simulink model "21-E"  (R2014a)
settings: Solver=FixedStepDiscrete  StartTime=0.0  StopTime=10.0  FixedStep=0.0005  RelTol=1e-3
undefined symbols (not defined in the file): add_k1_100, add_k2_100, ADDspeed, cal_acc_div, cal_acc_flo_add, cal_acc_min, cal_an_div, cal_an_min, cal_bre_div, cal_bre_en_add, cal_bre_flo_add, cal_bre_min, cal_conf_off, cal_conf_on, controller, ecucoder_acal, enres_on_add, enres_per_add
libraries: simulink x165, ec55xxlib x29
(part 6 of 6)

== system 21-E/run/ctrl/Subsystem1/control/Subsystem6 ==
  x1 : Inport
  x2 : Inport  Port=2
  x3 : Inport  Port=3
  x4 : Inport  Port=4
  k1 : Inport  Port=5
  k2 : Inport  Port=6
  Subsystem4 : Subsystem
  Subsystem5 : Subsystem
  alp1d : Outport
  alp2d : Outport  Port=2
  wires:
  Subsystem5/1(alp2d) -> alp2d/1
  x4/1 -> Subsystem5/2(x4)
  x2/1 -> Subsystem5/1(x2)
  k2/1 -> Subsystem5/3(k2)
  x3/1 -> Subsystem4/2(x3)
  k1/1 -> Subsystem4/3(k1)
  x1/1 -> Subsystem4/1(x1)
  Subsystem4/1(alp1d) -> alp1d/1

== system 21-E/run/ctrl/amk_tpostive1/差速/Subsystem1 ==
  vy : Inport
  yaw : Inport  Port=2
  ax : Inport  Port=3
  ay : Inport  Port=4
  Data Store Read : DataStoreRead  DataStoreName=ANGLE
  Data Store Read1 : DataStoreRead  DataStoreName=Vture
  Fz : Subsystem
  K : MATLAB Function  TreatAsAtomicUnit=on
  K1 : MATLAB Function  TreatAsAtomicUnit=on
  K2 : MATLAB Function  TreatAsAtomicUnit=on
  K3 : MATLAB Function  TreatAsAtomicUnit=on
  alp : Subsystem
  ctrl : Subsystem
  u3 : Outport
  w1 : Outport  Port=2
  w2 : Outport  Port=3
  w3 : Outport  Port=4
  w4 : Outport  Port=5
  tag scope: alp1l=global, alp1r=global, alp2l=global, alp2r=global, del=global, k1l=global, k1r=global, k2l=global, k2r=global, vx=global, vy=global, yaw=global
  wires:
  K3/1(k) -> [k2r]
  Fz/4(W2r) -> w4/1, K3/1(w)
  K2/1(k) -> [k2l]
  Fz/3(W2l) -> w3/1, K2/1(w)
  K1/1(k) -> [k1r]
  Fz/2(W1r) -> w2/1, K1/1(w)
  K/1(k) -> [k1l]
  Fz/1(W1l) -> w1/1, K/1(w)
  ay/1 -> Fz/2(ay)
  ax/1 -> Fz/1(ax)
  alp/4(alp_2R) -> [alp2r]
  alp/3(alp_2L) -> [alp2l]
  alp/2(alp_1R) -> [alp1r]
  alp/1(alp_1L) -> [alp1l]
  vy/1 -> [vy]
  yaw/1 -> [yaw]
  ctrl/1(u3) -> u3/1
  Data Store Read/1 -> [del]
  Data Store Read1/1 -> [vx]

== system 21-E/run/ctrl/amk_tpostive1/差速/Subsystem2 ==
  vx : Inport
  an : Inport  Port=2
  Add : Sum  Inputs=+-
  Add1 : Sum  Inputs=+-
  Add2 : Sum  Inputs=+-
  Constant : Constant  Value=0.01
  Constant1 : Constant  Value=0.01
  Constant2 : Constant  Value=0.01
  Delay : Delay  DelayLength=1  InitialCondition=0
  Delay1 : Delay  DelayLength=1  InitialCondition=0
  Delay2 : Delay  DelayLength=1  InitialCondition=0
  Product{,1..3} (4 alike) : Product  Inputs=*/
  Subsystem : Subsystem
  Trigonometric Function : Trigonometry  Operator=atan
  vy : Outport
  yaw : Outport  Port=2
  ax : Outport  Port=3
  ay : Outport  Port=4
  wires:
  Product/1 -> ay/1
  Add/1 -> Product/1
  Constant/1 -> Product/2
  Add1/1 -> Product1/1
  Constant1/1 -> Product1/2
  Product1/1 -> ax/1
  Delay1/1 -> Add1/2
  Delay/1 -> Add/2
  Subsystem/1(vy) -> Product3/1, vy/1, Delay/1, Add/1
  an/1 -> Subsystem/1(angle)
  vx/1 -> Product3/2, Delay1/1, Add1/1
  Add2/1 -> Product2/1
  Constant2/1 -> Product2/2
  Delay2/1 -> Add2/2
  Trigonometric Function/1 -> Add2/1, Delay2/1
  Product3/1 -> Trigonometric Function/1
  Product2/1 -> yaw/1

== system 21-E/run/ctrl/amk_tpostive1/限滑/V前 ==
  Data Store Read : DataStoreRead  DataStoreName=V1
  Data Store Read1 : DataStoreRead  DataStoreName=V2
  MinMax : MinMax  Function=max  Inputs=2
  Out1 : Outport
  wires:
  MinMax/1 -> Out1/1
  Data Store Read/1 -> MinMax/1
  Data Store Read1/1 -> MinMax/2

== system 21-E/run/ctrl/amk_tpostive1/限滑/V后 ==
  Data Store Read2 : DataStoreRead  DataStoreName=V3
  Data Store Read3 : DataStoreRead  DataStoreName=V4
  MinMax : MinMax  Function=max  Inputs=2
  Out1 : Outport
  wires:
  MinMax/1 -> Out1/1
  Data Store Read2/1 -> MinMax/1
  Data Store Read3/1 -> MinMax/2

== system 21-E/run/ctrl/amk_tpostive1/限滑/扭矩*PI1 ==
  扭矩 : Inport
  滑移率输入 : Inport  Port=2
  Constant2 : Constant
  Constant8 : Constant  Value=0.2
  Product : Product
  Saturation1 : Saturate  UpperLimit=1  LowerLimit=0
  Saturation2 : Saturate  UpperLimit=1  LowerLimit=0
  Saturation3 : Saturate  UpperLimit=1  LowerLimit=-1
  Saturation6 : Saturate  UpperLimit=2000  LowerLimit=0
  Sum1 : Sum  Inputs=|+-
  Sum4 : Sum  Inputs=|-+
  pid_discrete : Subsystem
  Out1 : Outport
  wires:
  Constant8/1 -> Sum4/2
  扭矩/1 -> Product/2
  Product/1 -> Saturation6/1
  Saturation6/1 -> Out1/1
  Saturation2/1 -> Product/1
  Saturation1/1 -> pid_discrete/2(y), Sum4/1
  Sum1/1 -> Saturation2/1
  Constant2/1 -> Sum1/1
  Sum4/1 -> Saturation3/1
  滑移率输入/1 -> Saturation1/1
  Saturation3/1 -> pid_discrete/1(err)
  pid_discrete/1(pid_out) -> Sum1/2  "pidhou"

== system 21-E/run/ctrl/amk_tpostive1/限滑/扭矩*PI2 ==
  滑移率输入 : Inport
  扭矩 : Inport  Port=2
  Constant2 : Constant
  Constant8 : Constant  Value=0.2
  Product : Product
  Saturation1 : Saturate  UpperLimit=1  LowerLimit=0
  Saturation2 : Saturate  UpperLimit=1  LowerLimit=0
  Saturation3 : Saturate  UpperLimit=1  LowerLimit=-1
  Saturation6 : Saturate  UpperLimit=2000  LowerLimit=0
  Sum1 : Sum  Inputs=|+-
  Sum4 : Sum  Inputs=|-+
  pid_discrete : Subsystem
  Out1 : Outport
  wires:
  扭矩/1 -> Product/2
  pid_discrete/1(pid_out) -> Sum1/2  "pidqian"
  Product/1 -> Saturation6/1
  Saturation6/1 -> Out1/1
  Saturation2/1 -> Product/1
  Saturation1/1 -> pid_discrete/2(y), Sum4/1
  Sum1/1 -> Saturation2/1
  Constant2/1 -> Sum1/1
  Sum4/1 -> Saturation3/1
  滑移率输入/1 -> Saturation1/1
  Constant8/1 -> Sum4/2
  Saturation3/1 -> pid_discrete/1(err)

== system 21-E/run/ctrl/amk_tpostive1/限滑/滑移率计算 ==
  V后 : Inport
  Add : Sum  Inputs=-+
  Constant : Constant  Value=0
  Data Store Read2 : DataStoreRead  DataStoreName=Vture
  Product1 : Product  Inputs=*/
  Switch2 : Switch  Criteria=u2 > Threshold  Threshold=500*1.88e-3
  Out : Outport
  wires:
  Data Store Read2/1 -> Add/1
  V后/1 -> Add/2, Switch2/2, Product1/2
  Add/1 -> Product1/1
  Product1/1 -> Switch2/1
  Constant/1 -> Switch2/3
  Switch2/1 -> Out/1

== system 21-E/run/ctrl/amk_tpostive1/限滑/滑移率计算1 ==
  V前 : Inport
  Add : Sum  Inputs=-+
  Constant : Constant  Value=0
  Data Store Read2 : DataStoreRead  DataStoreName=Vture
  Product1 : Product  Inputs=*/
  Switch2 : Switch  Criteria=u2 > Threshold  Threshold=500*1.88e-3
  Out : Outport
  wires:
  Data Store Read2/1 -> Add/1
  V前/1 -> Add/2, Switch2/2, Product1/2
  Add/1 -> Product1/1
  Product1/1 -> Switch2/1
  Constant/1 -> Switch2/3
  Switch2/1 -> Out/1

== system 21-E/run/ctrl/control/Subsystem6/Subsystem4 ==
  x1 : Inport
  x3 : Inport  Port=2
  k1 : Inport  Port=3
  Add : Sum  Inputs=+-
  Add1 : Sum  Inputs=+-
  Constant : Constant  Value=0.001
  Constant1 : Constant  Value=0.8
  Data Store Read : DataStoreRead  DataStoreName=a
  Divide : Product  Inputs=/*
  Gain : Gain  Gain=0.225
  Product : Product  Inputs=3
  Switch : Switch  Criteria=u2 > Threshold
  alp1d : Outport
  wires:
  Add/1 -> Product/2
  Add1/1 -> Divide/2
  Product/1 -> Add1/2
  Divide/1 -> alp1d/1
  Data Store Read/1 -> Add1/1
  Switch/1 -> Gain/1
  Constant/1 -> Switch/3
  x1/1 -> Product/3
  Constant1/1 -> Add/1
  Gain/1 -> Divide/1
  x3/1 -> Add/2, Switch/1, Switch/2
  k1/1 -> Product/1

== system 21-E/run/ctrl/control/Subsystem6/Subsystem5 ==
  x2 : Inport
  x4 : Inport  Port=2
  k2 : Inport  Port=3
  Add : Sum  Inputs=+-
  Add1 : Sum  Inputs=+-
  Constant : Constant  Value=0.001
  Constant1 : Constant  Value=0.8
  Data Store Read : DataStoreRead  DataStoreName=a
  Divide : Product  Inputs=/*
  Gain : Gain  Gain=0.225
  Product : Product  Inputs=3
  Switch : Switch  Criteria=u2 > Threshold
  alp2d : Outport
  wires:
  k2/1 -> Product/1
  x4/1 -> Switch/2, Switch/1, Add/2
  Gain/1 -> Divide/1
  Constant1/1 -> Add/1
  x2/1 -> Product/3
  Constant/1 -> Switch/3
  Switch/1 -> Gain/1
  Data Store Read/1 -> Add1/1
  Divide/1 -> alp2d/1
  Product/1 -> Add1/2
  Add1/1 -> Divide/2
  Add/1 -> Product/2

== system 21-E/run/ctrl/Subsystem1/control/Subsystem6/Subsystem4 ==
  x1 : Inport
  x3 : Inport  Port=2
  k1 : Inport  Port=3
  Add : Sum  Inputs=+-
  Add1 : Sum  Inputs=+-
  Constant : Constant  Value=0.001
  Constant1 : Constant  Value=0.8
  Data Store Read : DataStoreRead  DataStoreName=a
  Divide : Product  Inputs=/*
  Gain : Gain  Gain=0.225
  Product : Product  Inputs=3
  Switch : Switch  Criteria=u2 > Threshold
  alp1d : Outport
  wires:
  Add/1 -> Product/2
  Add1/1 -> Divide/2
  Product/1 -> Add1/2
  Divide/1 -> alp1d/1
  Data Store Read/1 -> Add1/1
  Switch/1 -> Gain/1
  Constant/1 -> Switch/3
  x1/1 -> Product/3
  Constant1/1 -> Add/1
  Gain/1 -> Divide/1
  x3/1 -> Add/2, Switch/1, Switch/2
  k1/1 -> Product/1

== system 21-E/run/ctrl/Subsystem1/control/Subsystem6/Subsystem5 ==
  x2 : Inport
  x4 : Inport  Port=2
  k2 : Inport  Port=3
  Add : Sum  Inputs=+-
  Add1 : Sum  Inputs=+-
  Constant : Constant  Value=0.001
  Constant1 : Constant  Value=0.8
  Data Store Read : DataStoreRead  DataStoreName=a
  Divide : Product  Inputs=/*
  Gain : Gain  Gain=0.225
  Product : Product  Inputs=3
  Switch : Switch  Criteria=u2 > Threshold
  alp2d : Outport
  wires:
  k2/1 -> Product/1
  x4/1 -> Switch/2, Switch/1, Add/2
  Gain/1 -> Divide/1
  Constant1/1 -> Add/1
  x2/1 -> Product/3
  Constant/1 -> Switch/3
  Switch/1 -> Gain/1
  Data Store Read/1 -> Add1/1
  Divide/1 -> alp2d/1
  Product/1 -> Add1/2
  Add1/1 -> Divide/2
  Add/1 -> Product/2

== system 21-E/run/ctrl/amk_tpostive1/差速/Subsystem1/Fz ==
  ax : Inport
  ay : Inport  Port=2
  Add : Sum
  L1 : Constant  Value=0.765
  L2 : Constant  Value=0.765
  M : Constant  Value=308
  Product : Product  Inputs=*/
  Subsystem : Subsystem
  Subsystem1 : Subsystem
  W1l : Outport
  W1r : Outport  Port=2
  W2l : Outport  Port=3
  W2r : Outport  Port=4
  wires:
  Subsystem1/2(w2r) -> W2r/1
  Subsystem1/1(w2l) -> W2l/1
  Subsystem/2(w1r) -> W1r/1
  Subsystem/1(w1l) -> W1l/1
  [ay] -> Subsystem1/4(ay)
  [ay] -> Subsystem/4(ay)
  [ax] -> Subsystem1/3(ax)
  [ax] -> Subsystem/3(ax)
  [L2] -> Subsystem/2(L2)
  Product/1 -> Subsystem/1(fac), Subsystem1/1(fac)
  [L1] -> Subsystem1/2(L1)
  ay/1 -> [ay]
  ax/1 -> [ax]
  M/1 -> Product/1
  Add/1 -> Product/2
  L2/1 -> Add/2, [L2]
  L1/1 -> Add/1, [L1]

== system 21-E/run/ctrl/amk_tpostive1/差速/Subsystem1/alp ==
  Constant{,2,4,6} (4 alike) : Constant  Value=0.765
  Constant{1,3,5,7} (4 alike) : Constant  Value=1.16
  MATLAB Function1 : MATLAB Function  TreatAsAtomicUnit=on
  MATLAB Function2 : MATLAB Function  TreatAsAtomicUnit=on
  MATLAB Function3 : MATLAB Function  TreatAsAtomicUnit=on
  MATLAB Function4 : MATLAB Function  TreatAsAtomicUnit=on
  Saturation{,1..3} (4 alike) : Saturate  UpperLimit=9/180*pi  LowerLimit=0
  alp_1L : Outport
  alp_1R : Outport  Port=2
  alp_2L : Outport  Port=3
  alp_2R : Outport  Port=4
  wires:
  Saturation3/1 -> alp_1L/1
  Saturation2/1 -> alp_2R/1
  Saturation1/1 -> alp_2L/1
  Saturation/1 -> alp_1R/1
  Constant6/1 -> MATLAB Function1/5(L1)
  Constant7/1 -> MATLAB Function1/6(D)
  Constant5/1 -> MATLAB Function4/5(D)
  Constant4/1 -> MATLAB Function4/4(L2)
  Constant2/1 -> MATLAB Function3/4(L2)
  Constant3/1 -> MATLAB Function3/5(D)
  Constant1/1 -> MATLAB Function2/6(D)
  MATLAB Function2/1(alp_1R) -> Saturation/1
  MATLAB Function4/1(alp_2R) -> Saturation2/1
  [vy] -> MATLAB Function1/2(vy)
  [yaw] -> MATLAB Function4/3(yaw)
  [del] -> MATLAB Function1/4(del)
  [vy] -> MATLAB Function2/2(vy)
  [del] -> MATLAB Function2/4(del)
  [vx] -> MATLAB Function2/1(v)
  MATLAB Function1/1(alp_1L) -> Saturation3/1
  [yaw] -> MATLAB Function3/3(yaw)
  [vx] -> MATLAB Function1/1(v)
  [yaw] -> MATLAB Function1/3(yaw)
  [vx] -> MATLAB Function4/1(v)
  [vy] -> MATLAB Function3/2(vy)
  [yaw] -> MATLAB Function2/3(yaw)
  MATLAB Function3/1(alp_2L) -> Saturation1/1
  [vy] -> MATLAB Function4/2(vy)
  Constant/1 -> MATLAB Function2/5(L1)
  [vx] -> MATLAB Function3/1(v)

== system 21-E/run/ctrl/amk_tpostive1/差速/Subsystem1/ctrl ==
  Manual Switch2 : ManualSwitch  CurrentSetting=0
  PID : Subsystem
  Subsystem1 : Subsystem
  rho : Subsystem
  slide : Subsystem
  u3 : Outport
  tag scope: e3=global, xd3=global
  wires:
  Manual Switch2/1 -> u3/1
  slide/1(u3) -> Manual Switch2/2
  PID/1(pid3) -> Manual Switch2/1
  rho/1(rho3) -> slide/3(rho3)
  [xd3] -> slide/2(x3)
  [e3] -> slide/1(e3)
  [yaw] -> PID/2(y3)
  [e3] -> PID/1(err3)
  Subsystem1/2(xd3) -> [xd3]
  Subsystem1/1(e3) -> [e3]
  [del] -> Subsystem1/3(del)
  [yaw] -> Subsystem1/2(yaw)
  [vx] -> Subsystem1/1(v)

== system 21-E/run/ctrl/amk_tpostive1/差速/Subsystem2/Subsystem ==
  angle : Inport
  Add : Sum
  Data Store Read2 : DataStoreRead  DataStoreName=V1
  Data Store Read3 : DataStoreRead  DataStoreName=V2
  Gain : Gain  Gain=0.5
  Product : Product
  Product1 : Product
  Trigonometric Function : Trigonometry
  Trigonometric Function1 : Trigonometry
  vy : Outport
  wires:
  Product/1 -> Add/1
  Trigonometric Function/1 -> Product/2
  Product1/1 -> Add/2
  Data Store Read3/1 -> Product1/1
  Data Store Read2/1 -> Product/1
  Add/1 -> Gain/1
  angle/1 -> Trigonometric Function1/1, Trigonometric Function/1
  Gain/1 -> vy/1
  Trigonometric Function1/1 -> Product1/2

== system 21-E/run/ctrl/amk_tpostive1/限滑/扭矩*PI1/pid_discrete ==
  err : Inport
  y : Inport  Port=2
  Add : Sum  Inputs=4
  Constant : Constant  Value=0.01
  Constant1 : Constant  Value=0.6
  Constant10 : Constant  Value=0
  Constant2 : Constant  Value=0.15
  Constant3 : Constant  Value=0.03
  Constant4 : Constant  Value=0.07
  Constant5 : Constant  Value=0
  Constant6 : Constant  Value=2000
  Constant7 : Constant  Value=0.6
  Constant8 : Constant  Value=0.03
  Constant9 : Constant  Value=0.01
  D : Subsystem
  I : Subsystem
  Memory : Memory  InheritSampleTime=on
  P : Subsystem
  dead_zone : Subsystem
  pid_out : Outport
  wires:
  Constant/1 -> dead_zone/2(err0)
  err/1 -> dead_zone/1(err_in)
  Add/1 -> pid_out/1, Memory/1
  Memory/1 -> Add/4, I/2(pid_in)
  P/1(Up) -> Add/1
  I/1(Ui) -> Add/2
  dead_zone/1(err_out) -> P/1(err), D/2(err), I/1(err)
  D/1(Ude) -> Add/3
  Constant1/1 -> P/2(kp)
  Constant4/1 -> I/5(ki)
  Constant6/1 -> I/7(up)
  Constant5/1 -> I/6(down)
  Constant2/1 -> I/3(sep)
  Constant3/1 -> I/4(len)
  y/1 -> D/1(y)
  Constant7/1 -> D/3(kp)
  Constant8/1 -> D/4(Td)
  Constant10/1 -> D/6(gama), D/7(zero)
  Constant9/1 -> D/5(T)

== system 21-E/run/ctrl/amk_tpostive1/限滑/扭矩*PI2/pid_discrete ==
  err : Inport
  y : Inport  Port=2
  Add : Sum  Inputs=4
  Constant : Constant  Value=0.01
  Constant1 : Constant  Value=0.6
  Constant10 : Constant  Value=0
  Constant2 : Constant  Value=0.15
  Constant3 : Constant  Value=0.03
  Constant4 : Constant  Value=0.07
  Constant5 : Constant  Value=0
  Constant6 : Constant  Value=2000
  Constant7 : Constant  Value=0.6
  Constant8 : Constant  Value=0.03
  Constant9 : Constant  Value=0.01
  D : Subsystem
  I : Subsystem
  Memory : Memory  InheritSampleTime=on
  P : Subsystem
  dead_zone : Subsystem
  pid_out : Outport
  wires:
  Constant/1 -> dead_zone/2(err0)
  err/1 -> dead_zone/1(err_in)
  Add/1 -> pid_out/1, Memory/1
  Memory/1 -> Add/4, I/2(pid_in)
  P/1(Up) -> Add/1
  I/1(Ui) -> Add/2
  dead_zone/1(err_out) -> P/1(err), D/2(err), I/1(err)
  D/1(Ude) -> Add/3
  Constant1/1 -> P/2(kp)
  Constant4/1 -> I/5(ki)
  Constant6/1 -> I/7(up)
  Constant5/1 -> I/6(down)
  Constant2/1 -> I/3(sep)
  Constant3/1 -> I/4(len)
  y/1 -> D/1(y)
  Constant7/1 -> D/3(kp)
  Constant8/1 -> D/4(Td)
  Constant10/1 -> D/6(gama), D/7(zero)
  Constant9/1 -> D/5(T)

== system 21-E/run/ctrl/amk_tpostive1/差速/Subsystem1/Fz/Subsystem ==
  fac : Inport
  L2 : Inport  Port=2
  ax : Inport  Port=3
  ay : Inport  Port=4
  Add : Sum  Inputs=+-
  Add1 : Sum  Inputs=+-
  Add2 : Sum  Inputs=2
  D : Constant  Value=1.18
  Demux : Demux  Outputs=2
  Gain : Gain  Gain=0.5
  Mux : Mux  Inputs=2
  Product : Product  Inputs=**/
  Product1 : Product
  g : Gain  Gain=9.8
  h1 : Gain  Gain=0.269
  h2 : Gain  Gain=0.269
  w1l : Outport
  w1r : Outport  Port=2
  wires:
  Demux/2 -> w1r/1
  Demux/1 -> w1l/1
  Product1/1 -> Demux/1
  fac/1 -> Product1/1
  Mux/1 -> Product1/2
  Add2/1 -> Mux/2
  Add1/1 -> Mux/1
  Product/1 -> Add1/2, Add2/2
  Gain/1 -> Add1/1, Add2/1
  D/1 -> Product/3
  ay/1 -> Product/2
  h2/1 -> Product/1
  Add/1 -> Gain/1
  h1/1 -> Add/2
  g/1 -> Add/1
  ax/1 -> h1/1
  L2/1 -> g/1, h2/1

== system 21-E/run/ctrl/amk_tpostive1/差速/Subsystem1/Fz/Subsystem1 ==
  fac : Inport
  L1 : Inport  Port=2
  ax : Inport  Port=3
  ay : Inport  Port=4
  Add : Sum  Inputs=2
  Add1 : Sum  Inputs=+-
  Add2 : Sum  Inputs=2
  D : Constant  Value=1.16
  Demux : Demux  Outputs=2
  Gain : Gain  Gain=0.5
  Mux : Mux  Inputs=2
  Product : Product  Inputs=**/
  Product1 : Product
  g : Gain  Gain=9.8
  h1 : Gain  Gain=0.269
  h2 : Gain  Gain=0.269
  w2l : Outport
  w2r : Outport  Port=2
  wires:
  L1/1 -> h2/1, g/1
  ax/1 -> h1/1
  g/1 -> Add/1
  h1/1 -> Add/2
  Add/1 -> Gain/1
  h2/1 -> Product/1
  ay/1 -> Product/2
  D/1 -> Product/3
  Gain/1 -> Add2/1, Add1/1
  Product/1 -> Add2/2, Add1/2
  Add1/1 -> Mux/1
  Add2/1 -> Mux/2
  Mux/1 -> Product1/2
  fac/1 -> Product1/1
  Product1/1 -> Demux/1
  Demux/1 -> w2l/1
  Demux/2 -> w2r/1

== system 21-E/run/ctrl/amk_tpostive1/差速/Subsystem1/ctrl/PID ==
  err3 : Inport
  y3 : Inport  Port=2
  pid_continuous2 : Subsystem
  pid3 : Outport
  wires:
  pid_continuous2/1(pid_out) -> pid3/1
  y3/1 -> pid_continuous2/2(y)
  err3/1 -> pid_continuous2/1(err)

== system 21-E/run/ctrl/amk_tpostive1/差速/Subsystem1/ctrl/Subsystem1 ==
  v : Inport
  yaw : Inport  Port=2
  del : Inport  Port=3
  Add2 : Sum  Inputs=+-
  Add3 : Sum  Inputs=2
  Constant1 : Constant
  K : Constant  Value=0.0002
  L_1 : Gain  Gain=1/(0.765+0.765)
  Math Function : Math  Operator=square  SaturateOnIntegerOverflow=on
  Product : Product  Inputs=**/
  Product1 : Product
  e3 : Outport
  xd3 : Outport  Port=2
  wires:
  yaw/1 -> Add2/2
  Constant1/1 -> Add3/2
  Math Function/1 -> Product1/1
  L_1/1 -> Product/1
  del/1 -> L_1/1
  Product1/1 -> Add3/1
  Add3/1 -> Product/3
  v/1 -> Math Function/1, Product/2
  K/1 -> Product1/2
  Add2/1 -> e3/1
  Product/1 -> Add2/1, xd3/1

== system 21-E/run/ctrl/amk_tpostive1/差速/Subsystem1/ctrl/rho ==
  Subsystem3 : Subsystem
  rho3 : Outport
  wires:
  Subsystem3/1(rho3) -> rho3/1
  [k1l] -> Subsystem3/1(k1)
  [k1r] -> Subsystem3/2(k2)
  [k2l] -> Subsystem3/3(k3)
  [k2r] -> Subsystem3/4(k4)
  [vx] -> Subsystem3/5(v)
  [yaw] -> Subsystem3/6(yaw)
  [vy] -> Subsystem3/7(vy)
  [del] -> Subsystem3/8(del)

== system 21-E/run/ctrl/amk_tpostive1/差速/Subsystem1/ctrl/slide ==
  e3 : Inport
  x3 : Inport  Port=2
  rho3 : Inport  Port=3
  Add3 : Sum  Inputs=3
  Derivative2 : Derivative
  MATLAB Function2 : MATLAB Function  TreatAsAtomicUnit=on
  Product2 : Product
  k3 : Gain  Gain=5
  u3 : Outport
  wires:
  x3/1 -> Derivative2/1
  Derivative2/1 -> Add3/1
  rho3/1 -> Product2/2
  e3/1 -> MATLAB Function2/1(e), k3/1
  Product2/1 -> Add3/3
  k3/1 -> Add3/2
  MATLAB Function2/1(s) -> Product2/1
  Add3/1 -> u3/1

== system 21-E/run/ctrl/amk_tpostive1/限滑/扭矩*PI1/pid_discrete/D ==
  y : Inport
  err : Inport  Port=2
  kp : Inport  Port=3
  Td : Inport  Port=4
  T : Inport  Port=5
  gama : Inport  Port=6
  zero : Inport  Port=7
  Add{,1..3} (4 alike) : Sum  Inputs=-+
  From : From  Commented=on  GotoTag=dy
  From1 : From  Commented=on  GotoTag=dym
  MATLAB Function1 : MATLAB Function  TreatAsAtomicUnit=on
  MATLAB Function2 : MATLAB Function  Commented=on  TreatAsAtomicUnit=on
  Product : Product  Commented=on  Inputs=**/
  Unit Delay{,1,3..5} (5 alike) : UnitDelay  SampleTime=-1
  Unit Delay2 : UnitDelay  Commented=on  SampleTime=-1
  Ude : Outport
  Udy : Outport  Port=2
  wires:
  y/1 -> Unit Delay/1, Add/2
  Unit Delay/1 -> Unit Delay1/1, Add1/2, Add/1
  Add/1 -> [dy]
  Unit Delay1/1 -> Add1/1
  Add1/1 -> [dym]
  Unit Delay2/1 -> MATLAB Function2/3(u_m)
  From/1 -> MATLAB Function2/1(y)
  From1/1 -> MATLAB Function2/2(y_m)
  Unit Delay3/1 -> MATLAB Function1/3(u_m)
  MATLAB Function1/1(u) -> Ude/1, Unit Delay3/1
  Add3/1 -> [dem]
  Unit Delay5/1 -> Add3/1
  Add2/1 -> [de]
  Unit Delay4/1 -> Add2/1, Add3/2, Unit Delay5/1
  err/1 -> Add2/2, Unit Delay4/1
  [de] -> MATLAB Function1/1(err)
  [dem] -> MATLAB Function1/2(err_m)
  kp/1 -> Product/1, MATLAB Function2/4(kp), MATLAB Function1/4(kp)
  gama/1 -> MATLAB Function2/6(gama), MATLAB Function1/7(gama)
  zero/1 -> MATLAB Function2/7(zero), MATLAB Function1/8(zero)
  Td/1 -> Product/2, MATLAB Function1/5(Td)
  T/1 -> Product/3, MATLAB Function1/6(T)
  Product/1 -> MATLAB Function2/5(kd)
  MATLAB Function2/1(u) -> Unit Delay2/1, Udy/1

== system 21-E/run/ctrl/amk_tpostive1/限滑/扭矩*PI1/pid_discrete/I ==
  err : Inport
  pid_in : Inport  Port=2
  sep : Inport  Port=3
  len : Inport  Port=4
  ki : Inport  Port=5
  down : Inport  Port=6
  up : Inport  Port=7
  Product1 : Product
  Product2 : Product
  Unit Delay : UnitDelay  SampleTime=-1
  f : MATLAB Function  TreatAsAtomicUnit=on
  sat : MATLAB Function  TreatAsAtomicUnit=on
  trape : MATLAB Function  TreatAsAtomicUnit=on
  Ui : Outport
  wires:
  err/1 -> Unit Delay/1, trape/1(err), sat/1(err), f/1(err)
  pid_in/1 -> sat/2(pid_in)
  trape/1(betay) -> Product1/1
  sat/1(anti) -> Product1/2
  Product1/1 -> Ui/1
  Unit Delay/1 -> trape/2(err_m)
  f/1(f) -> Product2/1
  ki/1 -> Product2/2
  Product2/1 -> trape/3(k)
  sep/1 -> f/2(sep)
  len/1 -> f/3(len)
  down/1 -> sat/3(down)
  up/1 -> sat/4(up)

== system 21-E/run/ctrl/amk_tpostive1/限滑/扭矩*PI1/pid_discrete/P ==
  err : Inport
  kp : Inport  Port=2
  Add : Sum  Inputs=+-
  Delay : Delay  DelayLength=1
  Product : Product
  Up : Outport
  wires:
  err/1 -> Add/1, Delay/1
  Delay/1 -> Add/2
  Add/1 -> Product/1
  Product/1 -> Up/1
  kp/1 -> Product/2

== system 21-E/run/ctrl/amk_tpostive1/限滑/扭矩*PI1/pid_discrete/dead_zone ==
  err_in : Inport
  err0 : Inport  Port=2
  MATLAB Function : MATLAB Function  TreatAsAtomicUnit=on
  err_out : Outport
  wires:
  err_in/1 -> MATLAB Function/1(err_in)
  MATLAB Function/1(err_out) -> err_out/1
  err0/1 -> MATLAB Function/2(err0)

== system 21-E/run/ctrl/amk_tpostive1/限滑/扭矩*PI2/pid_discrete/D ==
  y : Inport
  err : Inport  Port=2
  kp : Inport  Port=3
  Td : Inport  Port=4
  T : Inport  Port=5
  gama : Inport  Port=6
  zero : Inport  Port=7
  Add{,1..3} (4 alike) : Sum  Inputs=-+
  From : From  Commented=on  GotoTag=dy
  From1 : From  Commented=on  GotoTag=dym
  MATLAB Function1 : MATLAB Function  TreatAsAtomicUnit=on
  MATLAB Function2 : MATLAB Function  Commented=on  TreatAsAtomicUnit=on
  Product : Product  Commented=on  Inputs=**/
  Unit Delay{,1,3..5} (5 alike) : UnitDelay  SampleTime=-1
  Unit Delay2 : UnitDelay  Commented=on  SampleTime=-1
  Ude : Outport
  Udy : Outport  Port=2
  wires:
  y/1 -> Unit Delay/1, Add/2
  Unit Delay/1 -> Unit Delay1/1, Add1/2, Add/1
  Add/1 -> [dy]
  Unit Delay1/1 -> Add1/1
  Add1/1 -> [dym]
  Unit Delay2/1 -> MATLAB Function2/3(u_m)
  From/1 -> MATLAB Function2/1(y)
  From1/1 -> MATLAB Function2/2(y_m)
  Unit Delay3/1 -> MATLAB Function1/3(u_m)
  MATLAB Function1/1(u) -> Ude/1, Unit Delay3/1
  Add3/1 -> [dem]
  Unit Delay5/1 -> Add3/1
  Add2/1 -> [de]
  Unit Delay4/1 -> Add2/1, Add3/2, Unit Delay5/1
  err/1 -> Add2/2, Unit Delay4/1
  [de] -> MATLAB Function1/1(err)
  [dem] -> MATLAB Function1/2(err_m)
  kp/1 -> Product/1, MATLAB Function2/4(kp), MATLAB Function1/4(kp)
  gama/1 -> MATLAB Function2/6(gama), MATLAB Function1/7(gama)
  zero/1 -> MATLAB Function2/7(zero), MATLAB Function1/8(zero)
  Td/1 -> Product/2, MATLAB Function1/5(Td)
  T/1 -> Product/3, MATLAB Function1/6(T)
  Product/1 -> MATLAB Function2/5(kd)
  MATLAB Function2/1(u) -> Unit Delay2/1, Udy/1

== system 21-E/run/ctrl/amk_tpostive1/限滑/扭矩*PI2/pid_discrete/I ==
  err : Inport
  pid_in : Inport  Port=2
  sep : Inport  Port=3
  len : Inport  Port=4
  ki : Inport  Port=5
  down : Inport  Port=6
  up : Inport  Port=7
  Product1 : Product
  Product2 : Product
  Unit Delay : UnitDelay  SampleTime=-1
  f : MATLAB Function  TreatAsAtomicUnit=on
  sat : MATLAB Function  TreatAsAtomicUnit=on
  trape : MATLAB Function  TreatAsAtomicUnit=on
  Ui : Outport
  wires:
  err/1 -> Unit Delay/1, trape/1(err), sat/1(err), f/1(err)
  pid_in/1 -> sat/2(pid_in)
  trape/1(betay) -> Product1/1
  sat/1(anti) -> Product1/2
  Product1/1 -> Ui/1
  Unit Delay/1 -> trape/2(err_m)
  f/1(f) -> Product2/1
  ki/1 -> Product2/2
  Product2/1 -> trape/3(k)
  sep/1 -> f/2(sep)
  len/1 -> f/3(len)
  down/1 -> sat/3(down)
  up/1 -> sat/4(up)

== system 21-E/run/ctrl/amk_tpostive1/限滑/扭矩*PI2/pid_discrete/P ==
  err : Inport
  kp : Inport  Port=2
  Add : Sum  Inputs=+-
  Delay : Delay  DelayLength=1
  Product : Product
  Up : Outport
  wires:
  err/1 -> Add/1, Delay/1
  Delay/1 -> Add/2
  Add/1 -> Product/1
  Product/1 -> Up/1
  kp/1 -> Product/2

== system 21-E/run/ctrl/amk_tpostive1/限滑/扭矩*PI2/pid_discrete/dead_zone ==
  err_in : Inport
  err0 : Inport  Port=2
  MATLAB Function : MATLAB Function  TreatAsAtomicUnit=on
  err_out : Outport
  wires:
  err_in/1 -> MATLAB Function/1(err_in)
  MATLAB Function/1(err_out) -> err_out/1
  err0/1 -> MATLAB Function/2(err0)

== system 21-E/run/ctrl/amk_tpostive1/差速/Subsystem1/ctrl/PID/pid_continuous2 ==
  err : Inport
  y : Inport  Port=2
  Add : Sum  Inputs=3
  D : Subsystem
  I : Subsystem
  Memory : Memory
  P : Subsystem
  Product : Product  Inputs=*/
  Td : Constant  Value=0
  Ti : Constant
  dead_zone : Subsystem
  down : Constant  Value=0
  err0 : Constant  Value=0
  fore_switch : ManualSwitch  CurrentSetting=0
  gama : Constant  Value=0
  kp : Constant
  len : Constant  Value=0
  sep : Constant  Value=1e5
  up : Constant  Value=1e5
  zero : Constant  Value=0
  pid_out : Outport
  wires:
  err/1 -> dead_zone/1(err_in)
  P/1(P) -> Add/1
  I/1(I) -> Add/2
  Add/1 -> pid_out/1, Memory/1
  dead_zone/1(err_out) -> fore_switch/2, I/1(err), P/1(err)
  D/1(D) -> Add/3
  fore_switch/1 -> D/1(x)
  y/1 -> fore_switch/1
  Memory/1 -> I/2(pid_in)
  kp/1 -> [kp]
  Ti/1 -> [Ti]
  Td/1 -> [Td]
  [Ti] -> Product/2
  Product/1 -> I/3(ki)
  [kp] -> P/2(kp), Product/1, D/5(kp)
  err0/1 -> [err0]
  [err0] -> dead_zone/2(err0)
  down/1 -> [down]
  [down] -> I/4(down)
  up/1 -> [up]
  [up] -> I/5(up)
  sep/1 -> [sep]
  [sep] -> I/6(sep)
  len/1 -> [len]
  [len] -> I/7(len)
  gama/1 -> [gama]
  [gama] -> D/2(gama)
  [Td] -> D/3(Td)
  zero/1 -> [zero]
  [zero] -> D/4(zero)

== system 21-E/run/ctrl/amk_tpostive1/差速/Subsystem1/ctrl/rho/Subsystem3 ==
  k1 : Inport
  k2 : Inport  Port=2
  k3 : Inport  Port=3
  k4 : Inport  Port=4
  v : Inport  Port=5
  yaw : Inport  Port=6
  vy : Inport  Port=7
  del : Inport  Port=8
  2L1 : Gain  Gain=0.765*2
  Add1 : Sum  Inputs=+-
  Add2 : Sum  Inputs=+-
  Add{3..6} (4 alike) : Sum  Inputs=2
  D_2 : Gain  Gain=1.16*1.16
  Gain : Gain  Gain=0.5
  Gain1 : Gain  Gain=0.25
  Jz_1 : Gain  Gain=1/200
  L2 : Gain  Gain=0.765
  L2J_1 : Gain  Gain=0.765/200
  Math Function : Math  Operator=square  SaturateOnIntegerOverflow=on
  Math Function1 : Math  Operator=square  SaturateOnIntegerOverflow=on
  Product1 : Product
  Product2 : Product  Inputs=**/
  Product3 : Product
  fac : Constant  Value=pi*1.18/40
  rho3 : Outport
  wires:
  Jz_1/1 -> Product3/1
  Product3/1 -> Add3/1
  fac/1 -> Add6/2
  Add6/1 -> Product3/2
  2L1/1 -> Add6/1
  del/1 -> 2L1/1
  Gain/1 -> Jz_1/1
  Add5/1 -> Gain/1
  k2/1 -> Add5/2
  k1/1 -> Add5/1
  Math Function/1 -> Add2/1
  yaw/1 -> Math Function1/1, L2/1
  vy/1 -> Add1/2
  v/1 -> Product1/1, Math Function/1
  L2/1 -> Add1/1
  Gain1/1 -> Add2/2
  Math Function1/1 -> D_2/1
  D_2/1 -> Gain1/1
  Product1/1 -> Product2/2
  Add1/1 -> Product1/2
  Add2/1 -> Product2/3
  Add3/1 -> rho3/1
  Product2/1 -> Add3/2
  k3/1 -> Add4/1
  k4/1 -> Add4/2
  Add4/1 -> L2J_1/1
  L2J_1/1 -> Product2/1

== system 21-E/run/ctrl/amk_tpostive1/差速/Subsystem1/ctrl/PID/pid_continuous2/D ==
  x : Inport
  gama : Inport  Port=2
  Td : Inport  Port=3
  zero : Inport  Port=4
  kp : Inport  Port=5
  1st_order : Subsystem
  Add : Sum
  Derivative : Derivative
  Product{,1..3} (4 alike) : Product
  D : Outport
  wires:
  x/1 -> Product2/1, Derivative/1
  Product/1 -> Add/1
  Derivative/1 -> Product/2
  1st_order/1(y) -> Product3/1
  Add/1 -> 1st_order/2(x)
  Td/1 -> Product/1, Product1/2
  gama/1 -> Product1/1
  Product2/1 -> Add/2
  zero/1 -> Product2/2
  Product1/1 -> 1st_order/1(rTd)
  Product3/1 -> D/1
  kp/1 -> Product3/2

== system 21-E/run/ctrl/amk_tpostive1/差速/Subsystem1/ctrl/PID/pid_continuous2/I ==
  err : Inport
  pid_in : Inport  Port=2
  ki : Inport  Port=3
  down : Inport  Port=4
  up : Inport  Port=5
  sep : Inport  Port=6
  len : Inport  Port=7
  Integrator : Integrator
  MATLAB Function1 : MATLAB Function  TreatAsAtomicUnit=on
  Product : Product
  Product1 : Product
  f : MATLAB Function  TreatAsAtomicUnit=on
  I : Outport
  wires:
  err/1 -> f/1(err), MATLAB Function1/1(err)
  Product1/1 -> I/1
  Integrator/1 -> Product1/1
  pid_in/1 -> MATLAB Function1/2(in)
  MATLAB Function1/1(sat) -> Product/1
  Product/1 -> Integrator/1
  f/1(f) -> Product/2
  ki/1 -> Product1/2
  down/1 -> MATLAB Function1/3(down)
  up/1 -> MATLAB Function1/4(up)
  sep/1 -> f/2(sep)
  len/1 -> f/3(len)

== system 21-E/run/ctrl/amk_tpostive1/差速/Subsystem1/ctrl/PID/pid_continuous2/P ==
  err : Inport
  kp : Inport  Port=2
  Product : Product
  P : Outport
  wires:
  Product/1 -> P/1
  err/1 -> Product/1
  kp/1 -> Product/2

== system 21-E/run/ctrl/amk_tpostive1/差速/Subsystem1/ctrl/PID/pid_continuous2/dead_zone ==
  err_in : Inport
  err0 : Inport  Port=2
  MATLAB Function : MATLAB Function  TreatAsAtomicUnit=on
  err_out : Outport
  wires:
  err_in/1 -> MATLAB Function/1(err_in)
  MATLAB Function/1(err_out) -> err_out/1
  err0/1 -> MATLAB Function/2(err0)

== system 21-E/run/ctrl/amk_tpostive1/差速/Subsystem1/ctrl/PID/pid_continuous2/D/1st_order ==
  rTd : Inport
  x : Inport  Port=2
  Constant : Constant
  Integrator : Integrator
  Product : Product  Inputs=/*
  Sum : Sum  Inputs=|+-
  Switch : Switch  Criteria=u2 > Threshold
  Switch1 : Switch  Criteria=u2 > Threshold
  y : Outport
  wires:
  rTd/1 -> Switch1/2, Switch/1, Switch/2
  x/1 -> Switch1/3, Sum/1
  Product/1 -> Integrator/1
  Sum/1 -> Product/2
  Integrator/1 -> Switch1/1, Sum/2
  Switch/1 -> Product/1
  Constant/1 -> Switch/3
  Switch1/1 -> y/1

== matlab function 21-E/run/analog_acq/MATLAB Function ==
  data: x input; y input; d_ input; d output
function d = fcn(x,y,d_)
%#codegen
if (x && y)
    d=d_;
else
    d=x && y;
end

== matlab function 21-E/mot_trans/MATLAB Function ==
  data: s1 input; amk output; s2 input; s3 input; s4 input
function amk = fcn(s1,s2,s3,s4)
%#codegen
if (s1==s2 && s2==s3 && s3==s4)
    amk = s1;
else
    amk = uint16(0);
end

== matlab function 21-E/waiting/MATLAB Function1 ==
  data: en input; y output; count_whis data_store_memory; wait input
function y = fcn(en,wait)
%#codegen
if en == true
    y = false;
else
    y = wait;
end

== matlab function 21-E/run/analog_acq/MATLAB Function1 ==
  data: u input; y output; count_acc_sen data_store_memory
function y = fcn(u)
%#codegen
global count_acc_sen
if u==0
    count_acc_sen=0;
else
    count_acc_sen=count_acc_sen+1;
end
if count_acc_sen>=3
    a=1;
    count_acc_sen=3;
else
    a=0;
end
    
y = a;

== matlab function 21-E/run/analog_acq/MATLAB Function2 ==
  data: u input; y output; count_bre_sen data_store_memory
function y = fcn(u)
%#codegen
global count_bre_sen
if u==0
    count_bre_sen=0;
else
    count_bre_sen=count_bre_sen+1;
end
if count_bre_sen>=3
    a=1;
    count_bre_sen=3;
else
    a=0;
end
    
y = a;

== matlab function 21-E/waiting/MATLAB Function4 ==
  data: y output; count_en data_store_memory; can input; en input
function y = fcn(can,en)
%#codegen
if en == true && can == true
    y=false;
else
    y=en;
end

== matlab function 21-E/run/ctrl/Subsystem1/control/Subsystem1/MATLAB Function ==
  data: x input; s output; v input
function s  = fcn(x,v)
%#codegen
if x > 0
    s=1-v/x;
else
    s=0;
end

== matlab function 21-E/run/ctrl/Subsystem1/control/Subsystem1/MATLAB Function1 ==
  data: x input; s output; v input
function s  = fcn(x,v)
%#codegen
if x > 0
    s=1-v/x;
else
    s=0;
end

== matlab function 21-E/run/ctrl/Subsystem1/control/Subsystem2/MATLAB Function ==
  data: s input; phy output
function phy = fcn(s)
%#codegen

phy = 1.2801*(1-exp(-23.99*s))-0.52*s;

== matlab function 21-E/run/ctrl/Subsystem1/control/Subsystem2/MATLAB Function1 ==
  data: s input; phy output
function phy = fcn(s)
%#codegen

phy = 1.2801*(1-exp(-23.99*s))-0.52*s;

== matlab function 21-E/run/ctrl/Subsystem1/control/Subsystem3/MATLAB Function ==
  data: L1 input; W1 output; L2 input; M input; ah input; W2 output
function [W1,W2] = fcn(L1,L2,M,ah)
%#codegen
sl=2*(L1+L2);
W1=(9.8*L2 - ah)*M/sl;
W2=(9.8*L1 + ah)*M/sl;

== matlab function 21-E/run/ctrl/Subsystem1/Subsystem/MATLAB Function ==
  data: v input; T1 output; T1d input; T2d input; T2 output; slip_qian data_store_memory; slip_hou data_store_memory
function [T1,T2] = fcn(v,T1d,T2d)
%#codegen
global slip_qian
global slip_hou
if (v>0.5 && slip_qian > 0.08 && slip_hou > 0.08)
    T1=T1d;
    T2=T2d;
else
    T1=2000;
    T2=2000;
end

== matlab function 21-E/waiting/MATLAB Function2 ==
  data: u input; y output; count_can data_store_memory
function y = fcn(u)
%#codegen
global count_can
if u==0
    count_can=0;
else
    count_can=count_can+1;
end
if count_can>=200
    count_can=200;
    a=1;
else
    a=0;
end
y=a;

== matlab function 21-E/waiting/MATLAB Function3 ==
  data: u input; y output; count_whis data_store_memory; wait input
function y = fcn(u,wait)
%#codegen
global count_whis
if u==0
    count_whis=0;
else
    count_whis=count_whis+1;
end

if count_whis>=20
    count_whis=20;
    a=true;
else
    a=wait;
end
y=a;

== matlab function 21-E/waiting/MATLAB Function ==
  data: y output; count_en data_store_memory; u input; en input
function y = fcn(u,en)
%#codegen
global count_en
if u==1
    count_en=count_en+1;
else
    count_en=0;
end

if count_en>=260
    y= true ;
    count_en=260;
else
    y=en;
end

== matlab function 21-E/waiting/MATLAB Function5 ==
  data: en input; p output; count_whis data_store_memory; wait input; o output
function [p,o] = fcn(en,wait)
%#codegen
if en == true && wait==false
    p = 600000;
    o = 600000;
elseif wait == true && en==false
    p = 600000;
    o = 450000;
else
    p = 0;
    o = 0;
end

== matlab function 21-E/run/cal&con/MATLAB Function2 ==
  data: bre input; tri_lig output; count_bre_lig data_store_memory
function tri_lig = fcn(bre)
%#codegen
global count_bre_lig
if bre>=0.25
    count_bre_lig=count_bre_lig+1; 
else
   count_bre_lig=0;
end
if count_bre_lig>=60
    count_bre_lig=60;
    a=1;
else
    a=0;
end
    
tri_lig = a;

== matlab function 21-E/run/Subsystem/aim acceleration ==
  data: x input; g output
function g = f(x)
%#codegen
p1 =       68.79;
p2 =      -272.2;
p3 =       464.3;
p4 =      -436.7; 
p5 =       239.5; 
p6 =      -74.39; 
p7 =       12.04; 
p8 =    0.006415; 
p9 =    0.002764;
 g = p1*x^8 + p2*x^7 + p3*x^6 + p4*x^5 + p5*x^4 + p6*x^3 + p7*x^2 + p8*x + p9;

== matlab function 21-E/run/ctrl/Subsystem/MATLAB Function ==
  data: v input; reg output; bre input
function reg = fcn(v,bre)
%#codegen
if v>5 && bre>0.3 && bre<0.8
    reg=1;
else
    reg=0;
end

== matlab function 21-E/run/ctrl/MATLAB Function ==
  data: vm input; vf output; reg input
function vf = fcn(vm,reg)
%#codegen
if reg==1
    vf=0;
else
    vf=vm;
end

== matlab function 21-E/run/ctrl/amk_tpostive1/MATLAB Function ==
  data: v input; T output
function T = fcn(v)
%#codegen
if v<6000*1.88e-3
    T=2000;
elseif v>11000*1.88e-3
    T=900;
else
    T=1200;
end

== matlab function 21-E/run/ctrl/amk_tpostive1/限滑/扭矩*PI2/pid_discrete/D/MATLAB Function1 ==
  data: err input; u output; err_m input; u_m input; kp input; Td input; T input; gama input; zero input
function u = fcn(err,err_m,u_m,kp,Td,T,gama,zero)
a1=gama*Td/(gama*Td+T);
a2=kp*(Td+zero*T)/(gama*Td+T);
a3=kp*Td/(gama*Td+T);
u=a1*u_m+a2*err-a3*err_m;

== matlab function 21-E/run/ctrl/amk_tpostive1/限滑/扭矩*PI2/pid_discrete/D/MATLAB Function2 ==
  data: y input; u output; y_m input; u_m input; kp input; kd input; gama input; zero input
function u = fcn(y,y_m,u_m,kp,kd,gama,zero)
a4=gama*kd/(gama*kd+kp);
a5=(kd+zero*kp)/(gama*kd+kp);
a6=kd/(gama*kd+kp);
u=a4*u_m+a5*y-a6*y_m;

== matlab function 21-E/run/ctrl/amk_tpostive1/限滑/扭矩*PI2/pid_discrete/I/f ==
  data: err input; sep input; len input; f output
function f = fcn(err,sep,len)
if abs(err)<=sep
    f=1;
elseif abs(err)<sep+len
    f=1+(sep-abs(err))/len;
else
    f=0;
end

== matlab function 21-E/run/ctrl/amk_tpostive1/限滑/扭矩*PI2/pid_discrete/I/sat ==
  data: err input; anti output; pid_in input; down input; up input
function anti = fcn(err,pid_in,down,up)
if (pid_in < down && err<0)||(pid_in > up && err>0)
    anti=0;
else
    anti=1;
end

== matlab function 21-E/run/ctrl/amk_tpostive1/限滑/扭矩*PI2/pid_discrete/I/trape ==
  data: err input; err_m input; betay output; k input
function betay = fcn(err,err_m,k)
    betay=(err+err_m)/2*k;

== matlab function 21-E/run/ctrl/amk_tpostive1/限滑/扭矩*PI2/pid_discrete/dead_zone/MATLAB Function ==
  data: err_in input; err_out output; err0 input
function err_out = fcn(err_in,err0)
if abs(err_in)>err0
    err_out=err_in;
else
    err_out=0;
end

== matlab function 21-E/run/ctrl/amk_tpostive1/限滑/扭矩*PI1/pid_discrete/D/MATLAB Function1 ==
  data: err input; u output; err_m input; u_m input; kp input; Td input; T input; gama input; zero input
function u = fcn(err,err_m,u_m,kp,Td,T,gama,zero)
a1=gama*Td/(gama*Td+T);
a2=kp*(Td+zero*T)/(gama*Td+T);
a3=kp*Td/(gama*Td+T);
u=a1*u_m+a2*err-a3*err_m;

== matlab function 21-E/run/ctrl/amk_tpostive1/限滑/扭矩*PI1/pid_discrete/D/MATLAB Function2 ==
  data: y input; u output; y_m input; u_m input; kp input; kd input; gama input; zero input
function u = fcn(y,y_m,u_m,kp,kd,gama,zero)
a4=gama*kd/(gama*kd+kp);
a5=(kd+zero*kp)/(gama*kd+kp);
a6=kd/(gama*kd+kp);
u=a4*u_m+a5*y-a6*y_m;

== matlab function 21-E/run/ctrl/amk_tpostive1/限滑/扭矩*PI1/pid_discrete/I/f ==
  data: err input; sep input; len input; f output
function f = fcn(err,sep,len)
if abs(err)<=sep
    f=1;
elseif abs(err)<sep+len
    f=1+(sep-abs(err))/len;
else
    f=0;
end

== matlab function 21-E/run/ctrl/amk_tpostive1/限滑/扭矩*PI1/pid_discrete/I/sat ==
  data: err input; anti output; pid_in input; down input; up input
function anti = fcn(err,pid_in,down,up)
if (pid_in < down && err<0)||(pid_in > up && err>0)
    anti=0;
else
    anti=1;
end

== matlab function 21-E/run/ctrl/amk_tpostive1/限滑/扭矩*PI1/pid_discrete/I/trape ==
  data: err input; err_m input; betay output; k input
function betay = fcn(err,err_m,k)
    betay=(err+err_m)/2*k;

== matlab function 21-E/run/ctrl/amk_tpostive1/限滑/扭矩*PI1/pid_discrete/dead_zone/MATLAB Function ==
  data: err_in input; err_out output; err0 input
function err_out = fcn(err_in,err0)
if abs(err_in)>err0
    err_out=err_in;
else
    err_out=0;
end

== matlab function 21-E/run/ctrl/amk_tpostive1/差速/Subsystem1/K ==
  data: w input; k output
function k = fcn(w)

k =(8.487e-24*w.^9 - 5.859e-20*w.^8 + 1.686e-16*w.^7 ...
    - 2.619e-13*w.^6 + 2.377e-10*w.^5 - 1.271e-07*w.^4 ...
    + 3.8e-05*w.^3 - 0.005955*w.^2 + 1.493*w - 0.2143)*180/pi;

== matlab function 21-E/run/ctrl/amk_tpostive1/差速/Subsystem1/K1 ==
  data: w input; k output
function k = fcn(w)

k =(8.487e-24*w.^9 - 5.859e-20*w.^8 + 1.686e-16*w.^7 ...
    - 2.619e-13*w.^6 + 2.377e-10*w.^5 - 1.271e-07*w.^4 ...
    + 3.8e-05*w.^3 - 0.005955*w.^2 + 1.493*w - 0.2143)*180/pi;

== matlab function 21-E/run/ctrl/amk_tpostive1/差速/Subsystem1/K2 ==
  data: w input; k output
function k = fcn(w)

k =(8.487e-24*w.^9 - 5.859e-20*w.^8 + 1.686e-16*w.^7 ...
    - 2.619e-13*w.^6 + 2.377e-10*w.^5 - 1.271e-07*w.^4 ...
    + 3.8e-05*w.^3 - 0.005955*w.^2 + 1.493*w - 0.2143)*180/pi;

== matlab function 21-E/run/ctrl/amk_tpostive1/差速/Subsystem1/K3 ==
  data: w input; k output
function k = fcn(w)

k =(8.487e-24*w.^9 - 5.859e-20*w.^8 + 1.686e-16*w.^7 ...
    - 2.619e-13*w.^6 + 2.377e-10*w.^5 - 1.271e-07*w.^4 ...
    + 3.8e-05*w.^3 - 0.005955*w.^2 + 1.493*w - 0.2143)*180/pi;

== matlab function 21-E/run/ctrl/amk_tpostive1/差速/Subsystem1/alp/MATLAB Function1 ==
  data: v input; alp_1L output; vy input; yaw input; del input; L1 input; D input
function alp_1L = fcn(v,vy,yaw,del,L1,D)

alp_1L = del-atan((vy+yaw*L1)/(v-yaw*D/2));

== matlab function 21-E/run/ctrl/amk_tpostive1/差速/Subsystem1/alp/MATLAB Function2 ==
  data: v input; alp_1R output; vy input; yaw input; del input; L1 input; D input
function alp_1R = fcn(v,vy,yaw,del,L1,D)

alp_1R = del-atan((vy+yaw*L1)/(v+yaw*D/2));

== matlab function 21-E/run/ctrl/amk_tpostive1/差速/Subsystem1/alp/MATLAB Function3 ==
  data: v input; alp_2L output; vy input; yaw input; L2 input; D input
function alp_2L = fcn(v,vy,yaw,L2,D)

alp_2L = atan((yaw*L2-vy)/(v-yaw*D/2));

== matlab function 21-E/run/ctrl/amk_tpostive1/差速/Subsystem1/alp/MATLAB Function4 ==
  data: v input; alp_2R output; vy input; yaw input; L2 input; D input
function alp_2R = fcn(v,vy,yaw,L2,D)

alp_2R = atan((yaw*L2-vy)/(v+yaw*D/2));

== matlab function 21-E/run/ctrl/Subsystem2/MATLAB Function ==
  data: v input; T1 output; T1d input; T2d input; T2 output; slip_qian data_store_memory; slip_hou data_store_memory
function [T1,T2] = fcn(v,T1d,T2d)
%#codegen
global slip_qian
global slip_hou
if (v>0.5 && slip_qian > 0.08 && slip_hou > 0.08)
    T1=T1d;
    T2=T2d;
else
    T1=2000;
    T2=2000;
end

== matlab function 21-E/run/ctrl/control/Subsystem1/MATLAB Function ==
  data: x input; s output; v input
function s  = fcn(x,v)
%#codegen
if x > 0
    s=1-v/x;
else
    s=0;
end

== matlab function 21-E/run/ctrl/control/Subsystem1/MATLAB Function1 ==
  data: x input; s output; v input
function s  = fcn(x,v)
%#codegen
if x > 0
    s=1-v/x;
else
    s=0;
end

== matlab function 21-E/run/ctrl/control/Subsystem2/MATLAB Function ==
  data: s input; phy output
function phy = fcn(s)
%#codegen

phy = 1.2801*(1-exp(-23.99*s))-0.52*s;

== matlab function 21-E/run/ctrl/control/Subsystem2/MATLAB Function1 ==
  data: s input; phy output
function phy = fcn(s)
%#codegen

phy = 1.2801*(1-exp(-23.99*s))-0.52*s;

== matlab function 21-E/run/ctrl/control/Subsystem3/MATLAB Function ==
  data: L1 input; W1 output; L2 input; M input; ah input; W2 output
function [W1,W2] = fcn(L1,L2,M,ah)
%#codegen
sl=2*(L1+L2);
W1=(9.8*L2 - ah)*M/sl;
W2=(9.8*L1 + ah)*M/sl;

== matlab function 21-E/run/ctrl/amk_tpostive1/差速/Subsystem1/ctrl/PID/pid_continuous2/I/MATLAB Function1 ==
  data: err input; sat output; in input; down input; up input
function sat = fcn(err,in,down,up)
if (in>up && err>0)||(in<down && err<0)
    sat=0;
else
    sat=1;
end

== matlab function 21-E/run/ctrl/amk_tpostive1/差速/Subsystem1/ctrl/PID/pid_continuous2/I/f ==
  data: err input; sep input; len input; f output
function f = fcn(err,sep,len)
if abs(err)<=sep
    f=err;
elseif abs(err)<sep+len
    f=(1+(sep-abs(err))/len)*err;
else
    f=0;
end

== matlab function 21-E/run/ctrl/amk_tpostive1/差速/Subsystem1/ctrl/PID/pid_continuous2/dead_zone/MATLAB Function ==
  data: err_in input; err_out output; err0 input
function err_out = fcn(err_in,err0)
if abs(err_in)>err0
    err_out=err_in;
else
    err_out=0;
end

== matlab function 21-E/waiting1/MATLAB Function ==
  data: y output; count_en data_store_memory; u input; en input
function y = fcn(u,en)
%#codegen
global count_en
if u==1
    count_en=count_en+1;
else
    count_en=0;
end

if count_en>=260
    y= true ;
    count_en=260;
else
    y=en;
end

== matlab function 21-E/run/ctrl/amk_tpostive1/差速/Subsystem1/ctrl/slide/MATLAB Function2 ==
  data: e input; s output
function s = fcn(e)
d=abs(e);
if d<=1
    s=e;
else
    s=sign(e);
end

== matlab function 21-E/waiting1/MATLAB Function1 ==
  data: en input; y output; count_whis data_store_memory; wait input
function y = fcn(en,wait)
%#codegen
if en == true
    y = false;
else
    y = wait;
end

== matlab function 21-E/waiting1/MATLAB Function2 ==
  data: u input; y output; count_can data_store_memory
function y = fcn(u)
%#codegen
global count_can
if u==0
    count_can=0;
else
    count_can=count_can+1;
end
if count_can>=200
    count_can=200;
    a=1;
else
    a=0;
end
y=a;

== matlab function 21-E/waiting1/MATLAB Function3 ==
  data: u input; y output; count_whis data_store_memory; wait input
function y = fcn(u,wait)
%#codegen
global count_whis
if u==0
    count_whis=0;
else
    count_whis=count_whis+1;
end

if count_whis>=20
    count_whis=20;
    a=true;
else
    a=wait;
end
y=a;

== matlab function 21-E/waiting1/MATLAB Function4 ==
  data: y output; count_en data_store_memory; can input; en input
function y = fcn(can,en)
%#codegen
if en == true && can == true
    y=false;
else
    y=en;
end

== matlab function 21-E/waiting1/MATLAB Function5 ==
  data: en input; p output; count_whis data_store_memory; wait input; o output
function [p,o] = fcn(en,wait)
%#codegen
if en == true && wait==false
    p = 600000;
    o = 600000;
elseif wait == true && en==false
    p = 600000;
    o = 450000;
else
    p = 0;
    o = 0;
end
